simulink model "Par_model_sim_CHB7"  (R2023b)
settings: Solver=ode3  StartTime=0.0  StopTime=5  FixedStep=01e-6  RelTol=1e-3
InitFcn:
  | sysinit
values from neighbouring files (symbols this model uses):
  C = 0.0234    [sysinit.m]
  f_out = frequency_out_start : frequency_out_interval : frequency_out_end    [simout_chb_par.m]    (also in simout_chbjt_par.m = frequency_modulate_start : frequency_modulate_interval : fre)
  f_switch = 250    [sysinit.m]
  fn = 50    [sysinit.m]
  L = 0.002    [sysinit.m]
  L_1 = eps    [simout_chb_par.m]    (also in simout_chbjt_par.m; sysinit.m)
  L_ori = 0.02    [sysinit.m]
  L_sec = 0.06    [sysinit.m]
  m_par = modulate_radio_start : modulate_radio_interval : modulate_radio_end    [simout_chb_par.m]
  P0 = 8e6    (= 8000000)    [sysinit.m]
  R = 1.5    [sysinit.m]
  Source_Amp = 10000    [sysinit.m]
  st = 1e-6    (= 1e-06)    [sysinit.m]
  Td = 15e-7    (= 1.5e-06)    [sysinit.m]
  Ul_in = 1900    [sysinit.m]
libraries: spsSeriesRLCBranchLib x120, spsDiodeLib x45, spsIGBTLib x36, spsCurrentMeasurementLib x15, spsThreePhaseVIMeasurementLib x10, spsOnDelayLib x9, spsMultiWindingTransformerLib x9, spsUniversalBridgeLib x9, spsVoltageMeasurementLib x5, simulink x3, spsRMSLib x2, spsThreePhaseProgrammableVoltageSourceLib x1
(part 2 of 2)

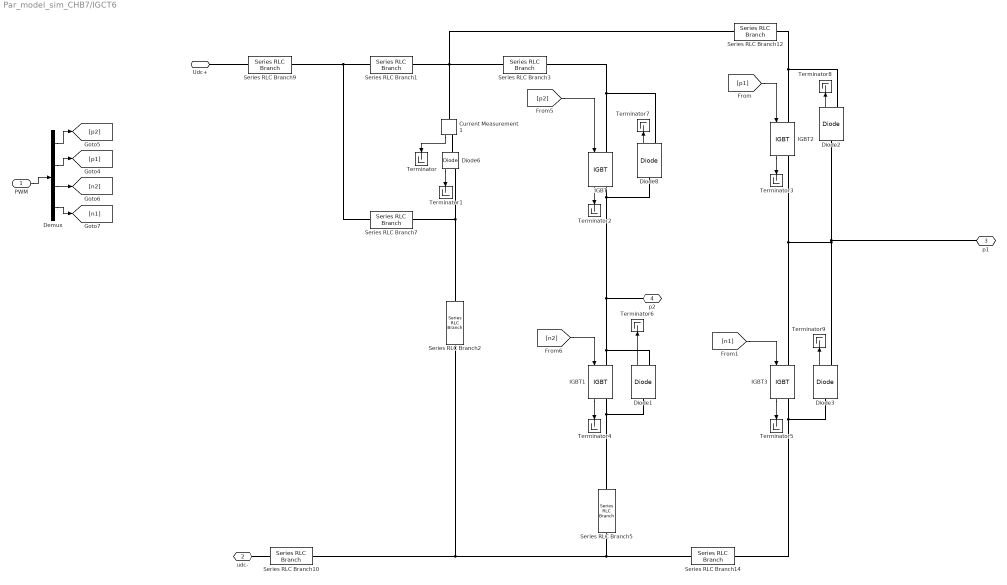
== system Par_model_sim_CHB7/IGCT6 ==
  PWM : Inport
  Current Measurement1 : spsCurrentMeasurementLib/Current Measurement  PhasorSimulation=off  OutputType=Complex  PSBequivalent=0
  Demux : Demux
  Diode{1..3,6,8} (5 alike) : spsDiodeLib/Diode  Ron=rto  Lon=0  Vf=vto  IC=0  UseSnubber=off  Rs=500  Cs=250e-9  Measurements=on
  IGBT{,1..3} (4 alike) : spsIGBTLib/IGBT  Ron=rt  Lon=0  Vf=vt  Tf=1e-6  Tt=2e-6  IC=0  Rs=1e5  Cs=inf  Measurements=on
  Series RLC Branch1 : spsSeriesRLCBranchLib/Series RLC Branch  LConnTagsString=__new0  RConnTagsString=__new0  BranchType=RL  Resistance=1e-5  Inductance=3.0E-6  SetiL0=off  InitialCurrent=0  Capacitance=1e-6  Setx0=off  InitialVoltage=0  Measurements=None
  Series RLC Branch10 : spsSeriesRLCBranchLib/Series RLC Branch  LConnTagsString=__new0  RConnTagsString=__new0  BranchType=L  Resistance=1  Inductance=0.4e-6  SetiL0=off  InitialCurrent=0  Capacitance=1e-6  Setx0=off  InitialVoltage=0  Measurements=None
  Series RLC Branch12 : spsSeriesRLCBranchLib/Series RLC Branch  LConnTagsString=__new0  RConnTagsString=__new0  BranchType=RL  Resistance=1e-5  Inductance=1E-9  SetiL0=off  InitialCurrent=0  Capacitance=1e-6  Setx0=off  InitialVoltage=0  Measurements=None
  Series RLC Branch14 : spsSeriesRLCBranchLib/Series RLC Branch  LConnTagsString=__new0  RConnTagsString=__new0  BranchType=L  Resistance=1  Inductance=1E-7  SetiL0=off  InitialCurrent=0  Capacitance=1e-6  Setx0=off  InitialVoltage=0  Measurements=None
  Series RLC Branch2 : spsSeriesRLCBranchLib/Series RLC Branch  LConnTagsString=__new0  RConnTagsString=__new0  BranchType=RC  Resistance=1e-5  Inductance=20e-6  SetiL0=off  InitialCurrent=0  Capacitance=17e-6  Setx0=off  InitialVoltage=0  Measurements=None
  Series RLC Branch3 : spsSeriesRLCBranchLib/Series RLC Branch  LConnTagsString=__new0  RConnTagsString=__new0  BranchType=RL  Resistance=1e-5  Inductance=1E-9  SetiL0=off  InitialCurrent=0  Capacitance=1e-6  Setx0=off  InitialVoltage=0  Measurements=None
  Series RLC Branch5 : spsSeriesRLCBranchLib/Series RLC Branch  LConnTagsString=__new0  RConnTagsString=__new0  BranchType=L  Resistance=1  Inductance=1E-7  SetiL0=off  InitialCurrent=0  Capacitance=1e-6  Setx0=off  InitialVoltage=0  Measurements=None
  Series RLC Branch7 : spsSeriesRLCBranchLib/Series RLC Branch  LConnTagsString=__new0  RConnTagsString=__new0  BranchType=RL  Resistance=0.6  Inductance=1e-6  SetiL0=off  InitialCurrent=0  Capacitance=1e-6  Setx0=off  InitialVoltage=0  Measurements=None
  Series RLC Branch9 : spsSeriesRLCBranchLib/Series RLC Branch  LConnTagsString=__new0  RConnTagsString=__new0  BranchType=L  Resistance=1  Inductance=0.4e-6  SetiL0=off  InitialCurrent=0  Capacitance=1e-6  Setx0=off  InitialVoltage=0  Measurements=None
  Terminator{,1..9} (10 alike) : Terminator
  Udc+ : PMIOPort  Side=Left
  udc- : PMIOPort  Port=2  Side=Left
  p1 : PMIOPort  Port=3  Side=Right
  p2 : PMIOPort  Port=4  Side=Right
  wires:
  Diode3/1 -> Terminator9/1
  IGBT3/1 -> Terminator5/1
  [n1] -> IGBT3/1
  IGBT1/1 -> Terminator4/1
  IGBT2/1 -> Terminator3/1
  IGBT/1 -> Terminator2/1
  [n2] -> IGBT1/1
  [p1] -> IGBT2/1
  Current Measurement1/1 -> Terminator/1
  Diode2/1 -> Terminator8/1
  [p2] -> IGBT/1
  Diode8/1 -> Terminator7/1
  Diode1/1 -> Terminator6/1
  Diode6/1 -> Terminator1/1
  Demux/3 -> [n2]
  PWM/1 -> Demux/1
  Demux/1 -> [p2]
  Demux/2 -> [p1]
  Demux/4 -> [n1]
  connections:
  Series RLC Branch10/LConn1 -- udc-/RConn1
  Series RLC Branch9/LConn1 -- Udc+/RConn1
  Diode6/RConn1 -- Series RLC Branch7/RConn1 -- Series RLC Branch2/LConn1
  Current Measurement1/LConn1 -- Series RLC Branch1/RConn1 -- Series RLC Branch3/LConn1 -- Series RLC Branch12/LConn1
  Diode3/LConn1 -- IGBT3/RConn1 -- Series RLC Branch14/RConn1
  Series RLC Branch3/RConn1 -- IGBT/LConn1 -- Diode8/RConn1
  Diode1/LConn1 -- Series RLC Branch5/RConn1 -- IGBT1/RConn1
  Current Measurement1/RConn1 -- Diode6/LConn1
  Diode2/RConn1 -- Series RLC Branch12/RConn1 -- IGBT2/LConn1
  p1/RConn1 -- Diode2/LConn1 -- Diode3/RConn1 -- IGBT3/LConn1 -- IGBT2/RConn1
  Series RLC Branch5/LConn1 -- Series RLC Branch14/LConn1 -- Series RLC Branch10/RConn1 -- Series RLC Branch2/RConn1
  Series RLC Branch1/LConn1 -- Series RLC Branch7/LConn1 -- Series RLC Branch9/RConn1
  p2/RConn1 -- IGBT1/LConn1 -- Diode1/RConn1 -- Diode8/LConn1 -- IGBT/RConn1

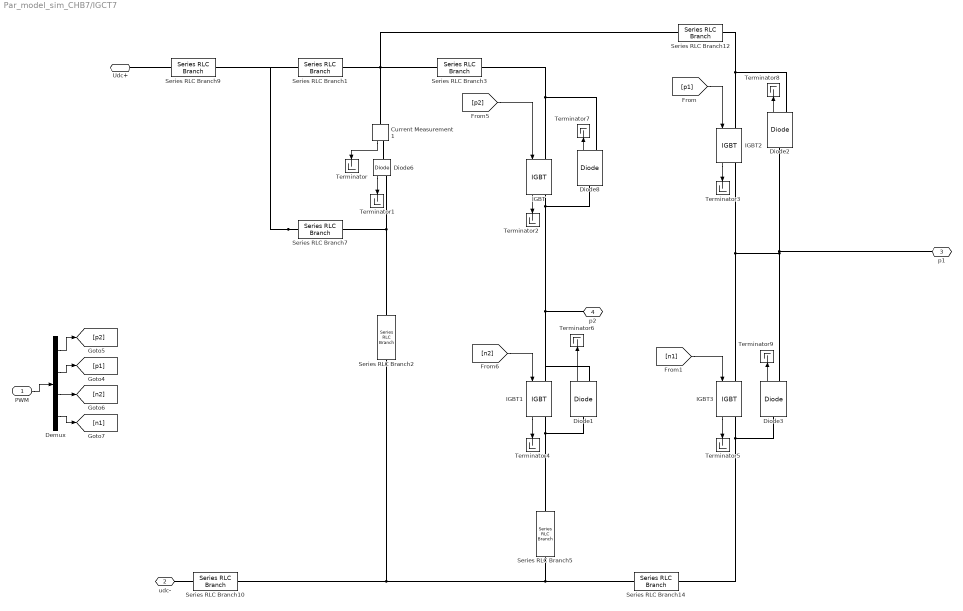
== system Par_model_sim_CHB7/IGCT7 ==
  PWM : Inport
  Current Measurement1 : spsCurrentMeasurementLib/Current Measurement  PhasorSimulation=off  OutputType=Complex  PSBequivalent=0
  Demux : Demux
  Diode{1..3,6,8} (5 alike) : spsDiodeLib/Diode  Ron=rto  Lon=0  Vf=vto  IC=0  UseSnubber=off  Rs=500  Cs=250e-9  Measurements=on
  IGBT{,1..3} (4 alike) : spsIGBTLib/IGBT  Ron=rt  Lon=0  Vf=vt  Tf=1e-6  Tt=2e-6  IC=0  Rs=1e5  Cs=inf  Measurements=on
  Series RLC Branch1 : spsSeriesRLCBranchLib/Series RLC Branch  LConnTagsString=__new0  RConnTagsString=__new0  BranchType=RL  Resistance=1e-5  Inductance=3.0E-6  SetiL0=off  InitialCurrent=0  Capacitance=1e-6  Setx0=off  InitialVoltage=0  Measurements=None
  Series RLC Branch10 : spsSeriesRLCBranchLib/Series RLC Branch  LConnTagsString=__new0  RConnTagsString=__new0  BranchType=L  Resistance=1  Inductance=0.4e-6  SetiL0=off  InitialCurrent=0  Capacitance=1e-6  Setx0=off  InitialVoltage=0  Measurements=None
  Series RLC Branch12 : spsSeriesRLCBranchLib/Series RLC Branch  LConnTagsString=__new0  RConnTagsString=__new0  BranchType=RL  Resistance=1e-5  Inductance=1E-9  SetiL0=off  InitialCurrent=0  Capacitance=1e-6  Setx0=off  InitialVoltage=0  Measurements=None
  Series RLC Branch14 : spsSeriesRLCBranchLib/Series RLC Branch  LConnTagsString=__new0  RConnTagsString=__new0  BranchType=L  Resistance=1  Inductance=1E-7  SetiL0=off  InitialCurrent=0  Capacitance=1e-6  Setx0=off  InitialVoltage=0  Measurements=None
  Series RLC Branch2 : spsSeriesRLCBranchLib/Series RLC Branch  LConnTagsString=__new0  RConnTagsString=__new0  BranchType=RC  Resistance=1e-5  Inductance=20e-6  SetiL0=off  InitialCurrent=0  Capacitance=17e-6  Setx0=off  InitialVoltage=0  Measurements=None
  Series RLC Branch3 : spsSeriesRLCBranchLib/Series RLC Branch  LConnTagsString=__new0  RConnTagsString=__new0  BranchType=RL  Resistance=1e-5  Inductance=1E-9  SetiL0=off  InitialCurrent=0  Capacitance=1e-6  Setx0=off  InitialVoltage=0  Measurements=None
  Series RLC Branch5 : spsSeriesRLCBranchLib/Series RLC Branch  LConnTagsString=__new0  RConnTagsString=__new0  BranchType=L  Resistance=1  Inductance=1E-7  SetiL0=off  InitialCurrent=0  Capacitance=1e-6  Setx0=off  InitialVoltage=0  Measurements=None
  Series RLC Branch7 : spsSeriesRLCBranchLib/Series RLC Branch  LConnTagsString=__new0  RConnTagsString=__new0  BranchType=RL  Resistance=0.6  Inductance=1e-6  SetiL0=off  InitialCurrent=0  Capacitance=1e-6  Setx0=off  InitialVoltage=0  Measurements=None
  Series RLC Branch9 : spsSeriesRLCBranchLib/Series RLC Branch  LConnTagsString=__new0  RConnTagsString=__new0  BranchType=L  Resistance=1  Inductance=0.4e-6  SetiL0=off  InitialCurrent=0  Capacitance=1e-6  Setx0=off  InitialVoltage=0  Measurements=None
  Terminator{,1..9} (10 alike) : Terminator
  Udc+ : PMIOPort  Side=Left
  udc- : PMIOPort  Port=2  Side=Left
  p1 : PMIOPort  Port=3  Side=Right
  p2 : PMIOPort  Port=4  Side=Right
  wires:
  Diode6/1 -> Terminator1/1
  Diode1/1 -> Terminator6/1
  Diode8/1 -> Terminator7/1
  PWM/1 -> Demux/1
  [p2] -> IGBT/1
  Diode2/1 -> Terminator8/1
  Current Measurement1/1 -> Terminator/1
  [p1] -> IGBT2/1
  [n2] -> IGBT1/1
  IGBT/1 -> Terminator2/1
  IGBT2/1 -> Terminator3/1
  Demux/4 -> [n1]
  Demux/3 -> [n2]
  Demux/2 -> [p1]
  IGBT1/1 -> Terminator4/1
  [n1] -> IGBT3/1
  IGBT3/1 -> Terminator5/1
  Diode3/1 -> Terminator9/1
  Demux/1 -> [p2]
  connections:
  IGBT/RConn1 -- Diode8/LConn1 -- p2/RConn1 -- Diode1/RConn1 -- IGBT1/LConn1
  Series RLC Branch7/LConn1 -- Series RLC Branch1/LConn1 -- Series RLC Branch9/RConn1
  Series RLC Branch14/LConn1 -- Series RLC Branch2/RConn1 -- Series RLC Branch10/RConn1 -- Series RLC Branch5/LConn1
  Diode2/LConn1 -- IGBT2/RConn1 -- IGBT3/LConn1 -- Diode3/RConn1 -- p1/RConn1
  Series RLC Branch12/RConn1 -- IGBT2/LConn1 -- Diode2/RConn1
  Current Measurement1/RConn1 -- Diode6/LConn1
  Series RLC Branch5/RConn1 -- Diode1/LConn1 -- IGBT1/RConn1
  IGBT/LConn1 -- Diode8/RConn1 -- Series RLC Branch3/RConn1
  IGBT3/RConn1 -- Diode3/LConn1 -- Series RLC Branch14/RConn1
  Series RLC Branch1/RConn1 -- Current Measurement1/LConn1 -- Series RLC Branch12/LConn1 -- Series RLC Branch3/LConn1
  Series RLC Branch7/RConn1 -- Diode6/RConn1 -- Series RLC Branch2/LConn1
  Series RLC Branch9/LConn1 -- Udc+/RConn1
  Series RLC Branch10/LConn1 -- udc-/RConn1

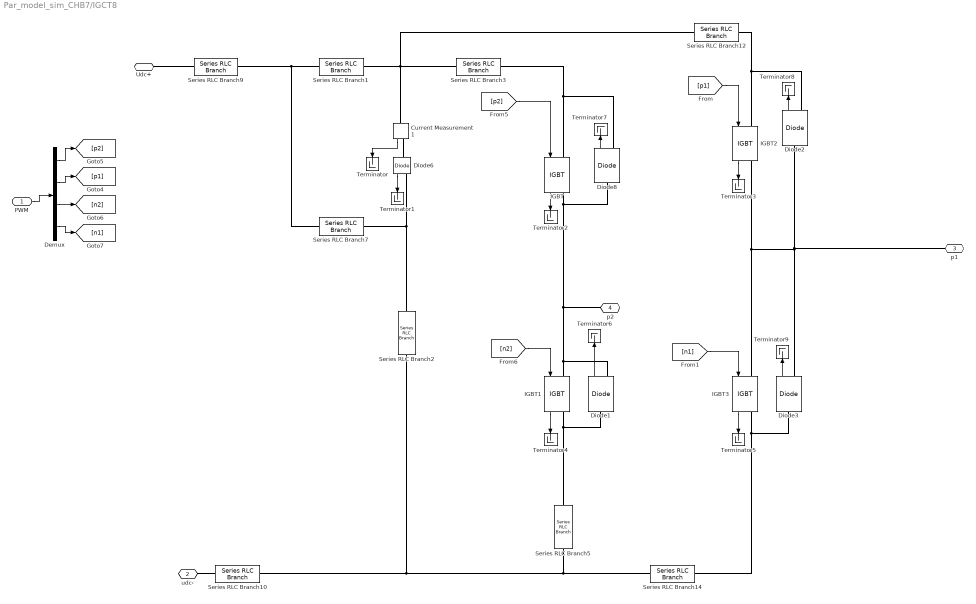
== system Par_model_sim_CHB7/IGCT8 ==
  PWM : Inport
  Current Measurement1 : spsCurrentMeasurementLib/Current Measurement  PhasorSimulation=off  OutputType=Complex  PSBequivalent=0
  Demux : Demux
  Diode{1..3,6,8} (5 alike) : spsDiodeLib/Diode  Ron=rto  Lon=0  Vf=vto  IC=0  UseSnubber=off  Rs=500  Cs=250e-9  Measurements=on
  IGBT{,1..3} (4 alike) : spsIGBTLib/IGBT  Ron=rt  Lon=0  Vf=vt  Tf=1e-6  Tt=2e-6  IC=0  Rs=1e5  Cs=inf  Measurements=on
  Series RLC Branch1 : spsSeriesRLCBranchLib/Series RLC Branch  LConnTagsString=__new0  RConnTagsString=__new0  BranchType=RL  Resistance=1e-5  Inductance=3.0E-6  SetiL0=off  InitialCurrent=0  Capacitance=1e-6  Setx0=off  InitialVoltage=0  Measurements=None
  Series RLC Branch10 : spsSeriesRLCBranchLib/Series RLC Branch  LConnTagsString=__new0  RConnTagsString=__new0  BranchType=L  Resistance=1  Inductance=0.4e-6  SetiL0=off  InitialCurrent=0  Capacitance=1e-6  Setx0=off  InitialVoltage=0  Measurements=None
  Series RLC Branch12 : spsSeriesRLCBranchLib/Series RLC Branch  LConnTagsString=__new0  RConnTagsString=__new0  BranchType=RL  Resistance=1e-5  Inductance=1E-9  SetiL0=off  InitialCurrent=0  Capacitance=1e-6  Setx0=off  InitialVoltage=0  Measurements=None
  Series RLC Branch14 : spsSeriesRLCBranchLib/Series RLC Branch  LConnTagsString=__new0  RConnTagsString=__new0  BranchType=L  Resistance=1  Inductance=1E-7  SetiL0=off  InitialCurrent=0  Capacitance=1e-6  Setx0=off  InitialVoltage=0  Measurements=None
  Series RLC Branch2 : spsSeriesRLCBranchLib/Series RLC Branch  LConnTagsString=__new0  RConnTagsString=__new0  BranchType=RC  Resistance=1e-5  Inductance=20e-6  SetiL0=off  InitialCurrent=0  Capacitance=17e-6  Setx0=off  InitialVoltage=0  Measurements=None
  Series RLC Branch3 : spsSeriesRLCBranchLib/Series RLC Branch  LConnTagsString=__new0  RConnTagsString=__new0  BranchType=RL  Resistance=1e-5  Inductance=1E-9  SetiL0=off  InitialCurrent=0  Capacitance=1e-6  Setx0=off  InitialVoltage=0  Measurements=None
  Series RLC Branch5 : spsSeriesRLCBranchLib/Series RLC Branch  LConnTagsString=__new0  RConnTagsString=__new0  BranchType=L  Resistance=1  Inductance=1E-7  SetiL0=off  InitialCurrent=0  Capacitance=1e-6  Setx0=off  InitialVoltage=0  Measurements=None
  Series RLC Branch7 : spsSeriesRLCBranchLib/Series RLC Branch  LConnTagsString=__new0  RConnTagsString=__new0  BranchType=RL  Resistance=0.6  Inductance=1e-6  SetiL0=off  InitialCurrent=0  Capacitance=1e-6  Setx0=off  InitialVoltage=0  Measurements=None
  Series RLC Branch9 : spsSeriesRLCBranchLib/Series RLC Branch  LConnTagsString=__new0  RConnTagsString=__new0  BranchType=L  Resistance=1  Inductance=0.4e-6  SetiL0=off  InitialCurrent=0  Capacitance=1e-6  Setx0=off  InitialVoltage=0  Measurements=None
  Terminator{,1..9} (10 alike) : Terminator
  Udc+ : PMIOPort  Side=Left
  udc- : PMIOPort  Port=2  Side=Left
  p1 : PMIOPort  Port=3  Side=Right
  p2 : PMIOPort  Port=4  Side=Right
  wires:
  Diode3/1 -> Terminator9/1
  IGBT3/1 -> Terminator5/1
  [n1] -> IGBT3/1
  IGBT1/1 -> Terminator4/1
  IGBT2/1 -> Terminator3/1
  IGBT/1 -> Terminator2/1
  [n2] -> IGBT1/1
  [p1] -> IGBT2/1
  Current Measurement1/1 -> Terminator/1
  Diode2/1 -> Terminator8/1
  [p2] -> IGBT/1
  Diode8/1 -> Terminator7/1
  Diode1/1 -> Terminator6/1
  Diode6/1 -> Terminator1/1
  Demux/3 -> [n2]
  PWM/1 -> Demux/1
  Demux/1 -> [p2]
  Demux/2 -> [p1]
  Demux/4 -> [n1]
  connections:
  Series RLC Branch10/LConn1 -- udc-/RConn1
  Series RLC Branch9/LConn1 -- Udc+/RConn1
  Diode6/RConn1 -- Series RLC Branch7/RConn1 -- Series RLC Branch2/LConn1
  Current Measurement1/LConn1 -- Series RLC Branch1/RConn1 -- Series RLC Branch3/LConn1 -- Series RLC Branch12/LConn1
  Diode3/LConn1 -- IGBT3/RConn1 -- Series RLC Branch14/RConn1
  Series RLC Branch3/RConn1 -- IGBT/LConn1 -- Diode8/RConn1
  Diode1/LConn1 -- Series RLC Branch5/RConn1 -- IGBT1/RConn1
  Current Measurement1/RConn1 -- Diode6/LConn1
  Diode2/RConn1 -- Series RLC Branch12/RConn1 -- IGBT2/LConn1
  p1/RConn1 -- Diode2/LConn1 -- Diode3/RConn1 -- IGBT3/LConn1 -- IGBT2/RConn1
  Series RLC Branch5/LConn1 -- Series RLC Branch14/LConn1 -- Series RLC Branch10/RConn1 -- Series RLC Branch2/RConn1
  Series RLC Branch1/LConn1 -- Series RLC Branch7/LConn1 -- Series RLC Branch9/RConn1
  p2/RConn1 -- IGBT1/LConn1 -- Diode1/RConn1 -- Diode8/LConn1 -- IGBT/RConn1

== system Par_model_sim_CHB7/IGCT9 ==
  PWM : Inport
  Current Measurement1 : spsCurrentMeasurementLib/Current Measurement  PhasorSimulation=off  OutputType=Complex  PSBequivalent=0
  Demux : Demux
  Diode{1..3,6,8} (5 alike) : spsDiodeLib/Diode  Ron=rto  Lon=0  Vf=vto  IC=0  UseSnubber=off  Rs=500  Cs=250e-9  Measurements=on
  IGBT{,1..3} (4 alike) : spsIGBTLib/IGBT  Ron=rt  Lon=0  Vf=vt  Tf=1e-6  Tt=2e-6  IC=0  Rs=1e5  Cs=inf  Measurements=on
  Series RLC Branch1 : spsSeriesRLCBranchLib/Series RLC Branch  LConnTagsString=__new0  RConnTagsString=__new0  BranchType=RL  Resistance=1e-5  Inductance=3.0E-6  SetiL0=off  InitialCurrent=0  Capacitance=1e-6  Setx0=off  InitialVoltage=0  Measurements=None
  Series RLC Branch10 : spsSeriesRLCBranchLib/Series RLC Branch  LConnTagsString=__new0  RConnTagsString=__new0  BranchType=L  Resistance=1  Inductance=0.4e-6  SetiL0=off  InitialCurrent=0  Capacitance=1e-6  Setx0=off  InitialVoltage=0  Measurements=None
  Series RLC Branch12 : spsSeriesRLCBranchLib/Series RLC Branch  LConnTagsString=__new0  RConnTagsString=__new0  BranchType=RL  Resistance=1e-5  Inductance=1E-9  SetiL0=off  InitialCurrent=0  Capacitance=1e-6  Setx0=off  InitialVoltage=0  Measurements=None
  Series RLC Branch14 : spsSeriesRLCBranchLib/Series RLC Branch  LConnTagsString=__new0  RConnTagsString=__new0  BranchType=L  Resistance=1  Inductance=1E-7  SetiL0=off  InitialCurrent=0  Capacitance=1e-6  Setx0=off  InitialVoltage=0  Measurements=None
  Series RLC Branch2 : spsSeriesRLCBranchLib/Series RLC Branch  LConnTagsString=__new0  RConnTagsString=__new0  BranchType=RC  Resistance=1e-5  Inductance=20e-6  SetiL0=off  InitialCurrent=0  Capacitance=17e-6  Setx0=off  InitialVoltage=0  Measurements=None
  Series RLC Branch3 : spsSeriesRLCBranchLib/Series RLC Branch  LConnTagsString=__new0  RConnTagsString=__new0  BranchType=RL  Resistance=1e-5  Inductance=1E-9  SetiL0=off  InitialCurrent=0  Capacitance=1e-6  Setx0=off  InitialVoltage=0  Measurements=None
  Series RLC Branch5 : spsSeriesRLCBranchLib/Series RLC Branch  LConnTagsString=__new0  RConnTagsString=__new0  BranchType=L  Resistance=1  Inductance=1E-7  SetiL0=off  InitialCurrent=0  Capacitance=1e-6  Setx0=off  InitialVoltage=0  Measurements=None
  Series RLC Branch7 : spsSeriesRLCBranchLib/Series RLC Branch  LConnTagsString=__new0  RConnTagsString=__new0  BranchType=RL  Resistance=0.6  Inductance=1e-6  SetiL0=off  InitialCurrent=0  Capacitance=1e-6  Setx0=off  InitialVoltage=0  Measurements=None
  Series RLC Branch9 : spsSeriesRLCBranchLib/Series RLC Branch  LConnTagsString=__new0  RConnTagsString=__new0  BranchType=L  Resistance=1  Inductance=0.4e-6  SetiL0=off  InitialCurrent=0  Capacitance=1e-6  Setx0=off  InitialVoltage=0  Measurements=None
  Terminator{,1..9} (10 alike) : Terminator
  Udc+ : PMIOPort  Side=Left
  udc- : PMIOPort  Port=2  Side=Left
  p1 : PMIOPort  Port=3  Side=Right
  p2 : PMIOPort  Port=4  Side=Right
  wires:
  Diode3/1 -> Terminator9/1
  IGBT3/1 -> Terminator5/1
  [n1] -> IGBT3/1
  IGBT1/1 -> Terminator4/1
  IGBT2/1 -> Terminator3/1
  IGBT/1 -> Terminator2/1
  [n2] -> IGBT1/1
  [p1] -> IGBT2/1
  Current Measurement1/1 -> Terminator/1
  Diode2/1 -> Terminator8/1
  [p2] -> IGBT/1
  Diode8/1 -> Terminator7/1
  Diode1/1 -> Terminator6/1
  Diode6/1 -> Terminator1/1
  Demux/3 -> [n2]
  PWM/1 -> Demux/1
  Demux/1 -> [p2]
  Demux/2 -> [p1]
  Demux/4 -> [n1]
  connections:
  Series RLC Branch10/LConn1 -- udc-/RConn1
  Series RLC Branch9/LConn1 -- Udc+/RConn1
  Diode6/RConn1 -- Series RLC Branch7/RConn1 -- Series RLC Branch2/LConn1
  Current Measurement1/LConn1 -- Series RLC Branch1/RConn1 -- Series RLC Branch3/LConn1 -- Series RLC Branch12/LConn1
  Diode3/LConn1 -- IGBT3/RConn1 -- Series RLC Branch14/RConn1
  Series RLC Branch3/RConn1 -- IGBT/LConn1 -- Diode8/RConn1
  Diode1/LConn1 -- Series RLC Branch5/RConn1 -- IGBT1/RConn1
  Current Measurement1/RConn1 -- Diode6/LConn1
  Diode2/RConn1 -- Series RLC Branch12/RConn1 -- IGBT2/LConn1
  p1/RConn1 -- Diode2/LConn1 -- Diode3/RConn1 -- IGBT3/LConn1 -- IGBT2/RConn1
  Series RLC Branch5/LConn1 -- Series RLC Branch14/LConn1 -- Series RLC Branch10/RConn1 -- Series RLC Branch2/RConn1
  Series RLC Branch1/LConn1 -- Series RLC Branch7/LConn1 -- Series RLC Branch9/RConn1
  p2/RConn1 -- IGBT1/LConn1 -- Diode1/RConn1 -- Diode8/LConn1 -- IGBT/RConn1

== system Par_model_sim_CHB7/LOAD ==
  Series RLC Branch1 : spsSeriesRLCBranchLib/Series RLC Branch  LConnTagsString=__new0  RConnTagsString=__new0  BranchType=RL  Resistance=R*1.5  Inductance=L*1.5  SetiL0=off  InitialCurrent=0  Capacitance=1e-6  Setx0=off  InitialVoltage=0  Measurements=None
  Series RLC Branch2 : spsSeriesRLCBranchLib/Series RLC Branch  LConnTagsString=__new0  RConnTagsString=__new0  BranchType=RL  Resistance=R*1.5  Inductance=L*1.5  SetiL0=off  InitialCurrent=0  Capacitance=1e-6  Setx0=off  InitialVoltage=0  Measurements=None
  Series RLC Branch7 : spsSeriesRLCBranchLib/Series RLC Branch  LConnTagsString=__new0  RConnTagsString=__new0  BranchType=RL  Resistance=R*1.5  Inductance=L*1.5  SetiL0=off  InitialCurrent=0  Capacitance=1e-6  Setx0=off  InitialVoltage=0  Measurements=None
  A : PMIOPort  Side=Left
  B : PMIOPort  Port=2  Side=Left
  C : PMIOPort  Port=3  Side=Left
  connections:
  Series RLC Branch7/RConn1 -- Series RLC Branch2/RConn1 -- Series RLC Branch1/RConn1
  Series RLC Branch2/LConn1 -- C/RConn1
  Series RLC Branch7/LConn1 -- A/RConn1
  Series RLC Branch1/LConn1 -- B/RConn1

== system Par_model_sim_CHB7/Subsystem ==
  Current Measurement : spsCurrentMeasurementLib/Current Measurement  PhasorSimulation=off  OutputType=Complex  PSBequivalent=0
  Voltage Measurement : spsVoltageMeasurementLib/Voltage Measurement  PhasorSimulation=off  OutputType=Complex  PSBequivalent=0
  + : PMIOPort  Side=Left
  - : PMIOPort  Port=2  Side=Left
  +OUT : PMIOPort  Port=3  Side=Right
  -OUT : PMIOPort  Port=4  Side=Right
  tag scope: Idc1=global, Udc=global
  wires:
  Voltage Measurement/1 -> [Udc]
  Current Measurement/1 -> [Idc1]
  connections:
  Voltage Measurement/LConn1 -- Current Measurement/LConn1 -- +/RConn1
  Voltage Measurement/LConn2 -- -OUT/RConn1 -- -/RConn1
  Current Measurement/RConn1 -- +OUT/RConn1

== system Par_model_sim_CHB7/Subsystem1 ==
  Current Measurement : spsCurrentMeasurementLib/Current Measurement  PhasorSimulation=off  OutputType=Complex  PSBequivalent=0
  Voltage Measurement : spsVoltageMeasurementLib/Voltage Measurement  PhasorSimulation=off  OutputType=Complex  PSBequivalent=0
  + : PMIOPort  Side=Left
  - : PMIOPort  Port=2  Side=Left
  +OUT : PMIOPort  Port=3  Side=Right
  -OUT : PMIOPort  Port=4  Side=Right
  tag scope: Idc2=global
  wires:
  Current Measurement/1 -> [Idc2]
  connections:
  Voltage Measurement/LConn1 -- +/RConn1 -- Current Measurement/LConn1
  Voltage Measurement/LConn2 -- -OUT/RConn1 -- -/RConn1
  Current Measurement/RConn1 -- +OUT/RConn1

== system Par_model_sim_CHB7/Subsystem2 ==
  Current Measurement : spsCurrentMeasurementLib/Current Measurement  PhasorSimulation=off  OutputType=Complex  PSBequivalent=0
  Voltage Measurement : spsVoltageMeasurementLib/Voltage Measurement  PhasorSimulation=off  OutputType=Complex  PSBequivalent=0
  + : PMIOPort  Side=Left
  - : PMIOPort  Port=2  Side=Left
  +OUT : PMIOPort  Port=3  Side=Right
  -OUT : PMIOPort  Port=4  Side=Right
  tag scope: Idc3=global
  wires:
  Current Measurement/1 -> [Idc3]
  connections:
  Voltage Measurement/LConn1 -- +/RConn1 -- Current Measurement/LConn1
  Voltage Measurement/LConn2 -- -OUT/RConn1 -- -/RConn1
  Current Measurement/RConn1 -- +OUT/RConn1

== system Par_model_sim_CHB7/Subsystem3 ==
  Series RLC Branch{1..9} (9 alike) : spsSeriesRLCBranchLib/Series RLC Branch  LConnTagsString=__new0  RConnTagsString=__new0  BranchType=L  Resistance=R*1.5  Inductance=L_in  SetiL0=off  InitialCurrent=0  Capacitance=1e-6  Setx0=off  InitialVoltage=0  Measurements=None
  Conn1 : PMIOPort  Side=Left
  Conn2 : PMIOPort  Port=2  Side=Right
  Conn3 : PMIOPort  Port=3  Side=Left
  Conn4 : PMIOPort  Port=4  Side=Right
  Conn5 : PMIOPort  Port=5  Side=Left
  Conn6 : PMIOPort  Port=6  Side=Right
  Conn7 : PMIOPort  Port=7  Side=Left
  Conn8 : PMIOPort  Port=8  Side=Right
  Conn9 : PMIOPort  Port=9  Side=Left
  Conn10 : PMIOPort  Port=10  Side=Right
  Conn11 : PMIOPort  Port=11  Side=Left
  Conn12 : PMIOPort  Port=12  Side=Right
  Conn13 : PMIOPort  Port=13  Side=Left
  Conn14 : PMIOPort  Port=14  Side=Right
  Conn15 : PMIOPort  Port=15  Side=Left
  Conn16 : PMIOPort  Port=16  Side=Right
  Conn17 : PMIOPort  Port=17  Side=Left
  Conn18 : PMIOPort  Port=18  Side=Right
  connections:
  Series RLC Branch3/RConn1 -- Conn8/RConn1
  Series RLC Branch3/LConn1 -- Conn7/RConn1
  Series RLC Branch7/LConn1 -- Conn1/RConn1
  Series RLC Branch7/RConn1 -- Conn2/RConn1
  Series RLC Branch1/LConn1 -- Conn3/RConn1
  Series RLC Branch2/LConn1 -- Conn5/RConn1
  Series RLC Branch4/LConn1 -- Conn9/RConn1
  Series RLC Branch5/LConn1 -- Conn11/RConn1
  Series RLC Branch4/RConn1 -- Conn10/RConn1
  Series RLC Branch1/RConn1 -- Conn4/RConn1
  Series RLC Branch5/RConn1 -- Conn12/RConn1
  Series RLC Branch9/LConn1 -- Conn17/RConn1
  Series RLC Branch8/LConn1 -- Conn15/RConn1
  Series RLC Branch6/RConn1 -- Conn14/RConn1
  Series RLC Branch9/RConn1 -- Conn18/RConn1
  Series RLC Branch8/RConn1 -- Conn16/RConn1
  Series RLC Branch6/LConn1 -- Conn13/RConn1
  Series RLC Branch2/RConn1 -- Conn6/RConn1

== system Par_model_sim_CHB7/Subsystem4 ==
  Series RLC Branch{1..9} (9 alike) : spsSeriesRLCBranchLib/Series RLC Branch  LConnTagsString=__new0  RConnTagsString=__new0  BranchType=L  Resistance=R*1.5  Inductance=L_in  SetiL0=off  InitialCurrent=0  Capacitance=1e-6  Setx0=off  InitialVoltage=0  Measurements=None
  Conn1 : PMIOPort  Side=Left
  Conn2 : PMIOPort  Port=2  Side=Right
  Conn3 : PMIOPort  Port=3  Side=Left
  Conn4 : PMIOPort  Port=4  Side=Right
  Conn5 : PMIOPort  Port=5  Side=Left
  Conn6 : PMIOPort  Port=6  Side=Right
  Conn7 : PMIOPort  Port=7  Side=Left
  Conn8 : PMIOPort  Port=8  Side=Right
  Conn9 : PMIOPort  Port=9  Side=Left
  Conn10 : PMIOPort  Port=10  Side=Right
  Conn11 : PMIOPort  Port=11  Side=Left
  Conn12 : PMIOPort  Port=12  Side=Right
  Conn13 : PMIOPort  Port=13  Side=Left
  Conn14 : PMIOPort  Port=14  Side=Right
  Conn15 : PMIOPort  Port=15  Side=Left
  Conn16 : PMIOPort  Port=16  Side=Right
  Conn17 : PMIOPort  Port=17  Side=Left
  Conn18 : PMIOPort  Port=18  Side=Right
  connections:
  Series RLC Branch2/RConn1 -- Conn6/RConn1
  Series RLC Branch6/LConn1 -- Conn13/RConn1
  Series RLC Branch8/RConn1 -- Conn16/RConn1
  Series RLC Branch9/RConn1 -- Conn18/RConn1
  Series RLC Branch6/RConn1 -- Conn14/RConn1
  Series RLC Branch8/LConn1 -- Conn15/RConn1
  Series RLC Branch9/LConn1 -- Conn17/RConn1
  Series RLC Branch5/RConn1 -- Conn12/RConn1
  Series RLC Branch1/RConn1 -- Conn4/RConn1
  Series RLC Branch4/RConn1 -- Conn10/RConn1
  Series RLC Branch5/LConn1 -- Conn11/RConn1
  Series RLC Branch4/LConn1 -- Conn9/RConn1
  Series RLC Branch2/LConn1 -- Conn5/RConn1
  Series RLC Branch1/LConn1 -- Conn3/RConn1
  Series RLC Branch7/RConn1 -- Conn2/RConn1
  Series RLC Branch7/LConn1 -- Conn1/RConn1
  Series RLC Branch3/LConn1 -- Conn7/RConn1
  Series RLC Branch3/RConn1 -- Conn8/RConn1

== system Par_model_sim_CHB7/Subsystem5 ==
  Series RLC Branch{1..9} (9 alike) : spsSeriesRLCBranchLib/Series RLC Branch  LConnTagsString=__new0  RConnTagsString=__new0  BranchType=L  Resistance=R*1.5  Inductance=L_in  SetiL0=off  InitialCurrent=0  Capacitance=1e-6  Setx0=off  InitialVoltage=0  Measurements=None
  Conn1 : PMIOPort  Side=Left
  Conn2 : PMIOPort  Port=2  Side=Right
  Conn3 : PMIOPort  Port=3  Side=Left
  Conn4 : PMIOPort  Port=4  Side=Right
  Conn5 : PMIOPort  Port=5  Side=Left
  Conn6 : PMIOPort  Port=6  Side=Right
  Conn7 : PMIOPort  Port=7  Side=Left
  Conn8 : PMIOPort  Port=8  Side=Right
  Conn9 : PMIOPort  Port=9  Side=Left
  Conn10 : PMIOPort  Port=10  Side=Right
  Conn11 : PMIOPort  Port=11  Side=Left
  Conn12 : PMIOPort  Port=12  Side=Right
  Conn13 : PMIOPort  Port=13  Side=Left
  Conn14 : PMIOPort  Port=14  Side=Right
  Conn15 : PMIOPort  Port=15  Side=Left
  Conn16 : PMIOPort  Port=16  Side=Right
  Conn17 : PMIOPort  Port=17  Side=Left
  Conn18 : PMIOPort  Port=18  Side=Right
  connections:
  Series RLC Branch3/RConn1 -- Conn8/RConn1
  Series RLC Branch3/LConn1 -- Conn7/RConn1
  Series RLC Branch7/LConn1 -- Conn1/RConn1
  Series RLC Branch7/RConn1 -- Conn2/RConn1
  Series RLC Branch1/LConn1 -- Conn3/RConn1
  Series RLC Branch2/LConn1 -- Conn5/RConn1
  Series RLC Branch4/LConn1 -- Conn9/RConn1
  Series RLC Branch5/LConn1 -- Conn11/RConn1
  Series RLC Branch4/RConn1 -- Conn10/RConn1
  Series RLC Branch1/RConn1 -- Conn4/RConn1
  Series RLC Branch5/RConn1 -- Conn12/RConn1
  Series RLC Branch9/LConn1 -- Conn17/RConn1
  Series RLC Branch8/LConn1 -- Conn15/RConn1
  Series RLC Branch6/RConn1 -- Conn14/RConn1
  Series RLC Branch9/RConn1 -- Conn18/RConn1
  Series RLC Branch8/RConn1 -- Conn16/RConn1
  Series RLC Branch6/LConn1 -- Conn13/RConn1
  Series RLC Branch2/RConn1 -- Conn6/RConn1

== system Par_model_sim_CHB7/Subsystem6 ==
  Multi-Winding Transformer10 : spsMultiWindingTransformerLib/Multi-Winding Transformer  LeftWindings=1  RightWindings=5  TappedWindings=no taps  NumberOfTaps=2  SetSaturation=off  Hysteresis=off  DataFile='hysteresis.mat'  Measurements=None  UNITS=pu  NominalPower=[P0 fn]  NominalVoltages="[ Source_Amp   (1-sin(10/180*pi)/sin(50/180*pi))*2*sin(50/180*pi)*Ul_in sin(10/180*pi)/sin(50/180*pi)*2*sin(50/180*pi)*Ul_in  Ul_in (1-sin(10/180*pi)/sin(50/180*pi))*2*sin(50/180*pi)*Ul_in sin(10/180*pi)/sin(50/180*pi)*2*sin(50/180*pi)*Ul_in]"  WindingResistances="[ 0.005   0.005 0.005 0.005  0.005  0.005]"  WindingInductances="[ L_ori*5  L_sec L_sec L_sec L_sec L_sec]/5"  Rm=50  Lm=50  Saturation=[ 0,0 ; 0.0024,1.2 ; 1.0,1.52 ]  SpecifyInitialFlux=off  InitialFlux=0  BreakLoop=off  DiscreteSolver=Trapezoidal iterative  DataType=off  TransfoNumber=1
      settings: LibrarySourceBlock=|
      | sps_lib/Power Grid Elements/Multi-Winding
      | Transformer
  Multi-Winding Transformer11 : spsMultiWindingTransformerLib/Multi-Winding Transformer  LeftWindings=1  RightWindings=5  TappedWindings=no taps  NumberOfTaps=2  SetSaturation=off  Hysteresis=off  DataFile='hysteresis.mat'  Measurements=None  UNITS=pu  NominalPower=[P0 fn]  NominalVoltages="[ Source_Amp   (1-sin(10/180*pi)/sin(50/180*pi))*2*sin(50/180*pi)*Ul_in sin(10/180*pi)/sin(50/180*pi)*2*sin(50/180*pi)*Ul_in  Ul_in (1-sin(10/180*pi)/sin(50/180*pi))*2*sin(50/180*pi)*Ul_in sin(10/180*pi)/sin(50/180*pi)*2*sin(50/180*pi)*Ul_in]"  WindingResistances="[ 0.005   0.005 0.005 0.005  0.005  0.005]"  WindingInductances="[ L_ori*5  L_sec L_sec L_sec L_sec L_sec]/5"  Rm=50  Lm=50  Saturation=[ 0,0 ; 0.0024,1.2 ; 1.0,1.52 ]  SpecifyInitialFlux=off  InitialFlux=0  BreakLoop=off  DiscreteSolver=Trapezoidal iterative  DataType=off  TransfoNumber=1
      settings: LibrarySourceBlock=|
      | sps_lib/Power Grid Elements/Multi-Winding
      | Transformer
  Multi-Winding Transformer9 : spsMultiWindingTransformerLib/Multi-Winding Transformer  LeftWindings=1  RightWindings=5  TappedWindings=no taps  NumberOfTaps=2  SetSaturation=off  Hysteresis=off  DataFile='hysteresis.mat'  Measurements=None  UNITS=pu  NominalPower=[P0 fn]  NominalVoltages="[ Source_Amp (1-sin(10/180*pi)/sin(50/180*pi))*2*sin(50/180*pi)*Ul_in sin(10/180*pi)/sin(50/180*pi)*2*sin(50/180*pi)*Ul_in  Ul_in (1-sin(10/180*pi)/sin(50/180*pi))*2*sin(50/180*pi)*Ul_in sin(10/180*pi)/sin(50/180*pi)*2*sin(50/180*pi)*Ul_in]"  WindingResistances="[ 0.005   0.005 0.005 0.005  0.005  0.005]"  WindingInductances="[ L_ori*5  L_sec L_sec L_sec L_sec L_sec]/5"  Rm=50  Lm=50  Saturation=[ 0,0 ; 0.0024,1.2 ; 1.0,1.52 ]  SpecifyInitialFlux=off  InitialFlux=0  BreakLoop=off  DiscreteSolver=Trapezoidal iterative  DataType=off  TransfoNumber=1
      settings: LibrarySourceBlock=|
      | sps_lib/Power Grid Elements/Multi-Winding
      | Transformer
  1+ : PMIOPort  Side=Left
  1+1 : PMIOPort  Port=2  Side=Left
  1+2 : PMIOPort  Port=3  Side=Left
  -20a : PMIOPort  Port=4  Side=Right
  -20b : PMIOPort  Port=5  Side=Right
  -20c : PMIOPort  Port=6  Side=Right
  0a : PMIOPort  Port=7  Side=Right
  0b : PMIOPort  Port=8  Side=Right
  0c : PMIOPort  Port=9  Side=Right
  +20a : PMIOPort  Port=10  Side=Right
  +20b : PMIOPort  Port=11  Side=Right
  +20c : PMIOPort  Port=12  Side=Right
  connections:
  Multi-Winding Transformer10/RConn9 -- +20b/RConn1
  Multi-Winding Transformer10/RConn5 -- 0b/RConn1
  Multi-Winding Transformer9/LConn1 -- 1+/RConn1
  Multi-Winding Transformer11/RConn9 -- +20c/RConn1
  +20a/RConn1 -- Multi-Winding Transformer9/RConn9
  Multi-Winding Transformer10/LConn1 -- 1+1/RConn1
  Multi-Winding Transformer9/RConn5 -- 0a/RConn1
  -20a/RConn1 -- Multi-Winding Transformer9/RConn3
  Multi-Winding Transformer11/RConn5 -- 0c/RConn1
  Multi-Winding Transformer11/LConn1 -- 1+2/RConn1
  Multi-Winding Transformer11/RConn3 -- -20c/RConn1
  Multi-Winding Transformer11/RConn2 -- Multi-Winding Transformer10/RConn4 -- Multi-Winding Transformer10/RConn1
  Multi-Winding Transformer10/RConn3 -- -20b/RConn1
  Multi-Winding Transformer11/RConn8 -- Multi-Winding Transformer9/RConn7 -- Multi-Winding Transformer9/RConn10
  Multi-Winding Transformer11/RConn4 -- Multi-Winding Transformer9/RConn2 -- Multi-Winding Transformer11/RConn1
  Multi-Winding Transformer10/RConn10 -- Multi-Winding Transformer9/RConn8 -- Multi-Winding Transformer10/RConn7
  Multi-Winding Transformer11/RConn6 -- Multi-Winding Transformer9/RConn6 -- Multi-Winding Transformer10/RConn6
  Multi-Winding Transformer10/RConn2 -- Multi-Winding Transformer9/RConn4 -- Multi-Winding Transformer9/RConn1
  Multi-Winding Transformer11/RConn10 -- Multi-Winding Transformer10/RConn8 -- Multi-Winding Transformer11/RConn7
  Multi-Winding Transformer11/LConn2 -- Multi-Winding Transformer9/LConn2 -- Multi-Winding Transformer10/LConn2

== system Par_model_sim_CHB7/Subsystem7 ==
  Multi-Winding Transformer10 : spsMultiWindingTransformerLib/Multi-Winding Transformer  LeftWindings=1  RightWindings=5  TappedWindings=no taps  NumberOfTaps=2  SetSaturation=off  Hysteresis=off  DataFile='hysteresis.mat'  Measurements=None  UNITS=pu  NominalPower=[P0 fn]  NominalVoltages="[ Source_Amp   (1-sin(10/180*pi)/sin(50/180*pi))*2*sin(50/180*pi)*Ul_in sin(10/180*pi)/sin(50/180*pi)*2*sin(50/180*pi)*Ul_in  Ul_in (1-sin(10/180*pi)/sin(50/180*pi))*2*sin(50/180*pi)*Ul_in sin(10/180*pi)/sin(50/180*pi)*2*sin(50/180*pi)*Ul_in]"  WindingResistances="[ 0.005   0.005 0.005 0.005  0.005  0.005]"  WindingInductances="[ L_ori*5  L_sec L_sec L_sec L_sec L_sec]/5"  Rm=50  Lm=50  Saturation=[ 0,0 ; 0.0024,1.2 ; 1.0,1.52 ]  SpecifyInitialFlux=off  InitialFlux=0  BreakLoop=off  DiscreteSolver=Trapezoidal iterative  DataType=off  TransfoNumber=1
      settings: LibrarySourceBlock=|
      | sps_lib/Power Grid Elements/Multi-Winding
      | Transformer
  Multi-Winding Transformer11 : spsMultiWindingTransformerLib/Multi-Winding Transformer  LeftWindings=1  RightWindings=5  TappedWindings=no taps  NumberOfTaps=2  SetSaturation=off  Hysteresis=off  DataFile='hysteresis.mat'  Measurements=None  UNITS=pu  NominalPower=[P0 fn]  NominalVoltages="[ Source_Amp   (1-sin(10/180*pi)/sin(50/180*pi))*2*sin(50/180*pi)*Ul_in sin(10/180*pi)/sin(50/180*pi)*2*sin(50/180*pi)*Ul_in  Ul_in (1-sin(10/180*pi)/sin(50/180*pi))*2*sin(50/180*pi)*Ul_in sin(10/180*pi)/sin(50/180*pi)*2*sin(50/180*pi)*Ul_in]"  WindingResistances="[ 0.005   0.005 0.005 0.005  0.005  0.005]"  WindingInductances="[ L_ori*5  L_sec L_sec L_sec L_sec L_sec]/5"  Rm=50  Lm=50  Saturation=[ 0,0 ; 0.0024,1.2 ; 1.0,1.52 ]  SpecifyInitialFlux=off  InitialFlux=0  BreakLoop=off  DiscreteSolver=Trapezoidal iterative  DataType=off  TransfoNumber=1
      settings: LibrarySourceBlock=|
      | sps_lib/Power Grid Elements/Multi-Winding
      | Transformer
  Multi-Winding Transformer9 : spsMultiWindingTransformerLib/Multi-Winding Transformer  LeftWindings=1  RightWindings=5  TappedWindings=no taps  NumberOfTaps=2  SetSaturation=off  Hysteresis=off  DataFile='hysteresis.mat'  Measurements=None  UNITS=pu  NominalPower=[P0 fn]  NominalVoltages="[ Source_Amp (1-sin(10/180*pi)/sin(50/180*pi))*2*sin(50/180*pi)*Ul_in sin(10/180*pi)/sin(50/180*pi)*2*sin(50/180*pi)*Ul_in  Ul_in (1-sin(10/180*pi)/sin(50/180*pi))*2*sin(50/180*pi)*Ul_in sin(10/180*pi)/sin(50/180*pi)*2*sin(50/180*pi)*Ul_in]"  WindingResistances="[ 0.005   0.005 0.005 0.005  0.005  0.005]"  WindingInductances="[ L_ori*5  L_sec L_sec L_sec L_sec L_sec]/5"  Rm=50  Lm=50  Saturation=[ 0,0 ; 0.0024,1.2 ; 1.0,1.52 ]  SpecifyInitialFlux=off  InitialFlux=0  BreakLoop=off  DiscreteSolver=Trapezoidal iterative  DataType=off  TransfoNumber=1
      settings: LibrarySourceBlock=|
      | sps_lib/Power Grid Elements/Multi-Winding
      | Transformer
  1+ : PMIOPort  Side=Left
  1+1 : PMIOPort  Port=2  Side=Left
  1+2 : PMIOPort  Port=3  Side=Left
  -20a : PMIOPort  Port=4  Side=Right
  -20b : PMIOPort  Port=5  Side=Right
  -20c : PMIOPort  Port=6  Side=Right
  0a : PMIOPort  Port=7  Side=Right
  0b : PMIOPort  Port=8  Side=Right
  0c : PMIOPort  Port=9  Side=Right
  +20a : PMIOPort  Port=10  Side=Right
  +20b : PMIOPort  Port=11  Side=Right
  +20c : PMIOPort  Port=12  Side=Right
  connections:
  Multi-Winding Transformer10/LConn2 -- Multi-Winding Transformer9/LConn2 -- Multi-Winding Transformer11/LConn2
  Multi-Winding Transformer11/RConn7 -- Multi-Winding Transformer10/RConn8 -- Multi-Winding Transformer11/RConn10
  Multi-Winding Transformer9/RConn1 -- Multi-Winding Transformer9/RConn4 -- Multi-Winding Transformer10/RConn2
  Multi-Winding Transformer10/RConn6 -- Multi-Winding Transformer9/RConn6 -- Multi-Winding Transformer11/RConn6
  Multi-Winding Transformer10/RConn7 -- Multi-Winding Transformer9/RConn8 -- Multi-Winding Transformer10/RConn10
  Multi-Winding Transformer11/RConn1 -- Multi-Winding Transformer9/RConn2 -- Multi-Winding Transformer11/RConn4
  Multi-Winding Transformer9/RConn10 -- Multi-Winding Transformer9/RConn7 -- Multi-Winding Transformer11/RConn8
  Multi-Winding Transformer10/RConn3 -- -20b/RConn1
  Multi-Winding Transformer10/RConn1 -- Multi-Winding Transformer10/RConn4 -- Multi-Winding Transformer11/RConn2
  Multi-Winding Transformer11/RConn3 -- -20c/RConn1
  Multi-Winding Transformer11/LConn1 -- 1+2/RConn1
  Multi-Winding Transformer11/RConn5 -- 0c/RConn1
  -20a/RConn1 -- Multi-Winding Transformer9/RConn3
  Multi-Winding Transformer9/RConn5 -- 0a/RConn1
  Multi-Winding Transformer10/LConn1 -- 1+1/RConn1
  +20a/RConn1 -- Multi-Winding Transformer9/RConn9
  Multi-Winding Transformer11/RConn9 -- +20c/RConn1
  Multi-Winding Transformer9/LConn1 -- 1+/RConn1
  Multi-Winding Transformer10/RConn5 -- 0b/RConn1
  Multi-Winding Transformer10/RConn9 -- +20b/RConn1

== system Par_model_sim_CHB7/Subsystem8 ==
  Multi-Winding Transformer10 : spsMultiWindingTransformerLib/Multi-Winding Transformer  LeftWindings=1  RightWindings=5  TappedWindings=no taps  NumberOfTaps=2  SetSaturation=off  Hysteresis=off  DataFile='hysteresis.mat'  Measurements=None  UNITS=pu  NominalPower=[P0 fn]  NominalVoltages="[ Source_Amp   (1-sin(10/180*pi)/sin(50/180*pi))*2*sin(50/180*pi)*Ul_in sin(10/180*pi)/sin(50/180*pi)*2*sin(50/180*pi)*Ul_in  Ul_in (1-sin(10/180*pi)/sin(50/180*pi))*2*sin(50/180*pi)*Ul_in sin(10/180*pi)/sin(50/180*pi)*2*sin(50/180*pi)*Ul_in]"  WindingResistances="[ 0.005   0.005 0.005 0.005  0.005  0.005]"  WindingInductances="[ L_ori*5  L_sec L_sec L_sec L_sec L_sec]/5"  Rm=50  Lm=50  Saturation=[ 0,0 ; 0.0024,1.2 ; 1.0,1.52 ]  SpecifyInitialFlux=off  InitialFlux=0  BreakLoop=off  DiscreteSolver=Trapezoidal iterative  DataType=off  TransfoNumber=1
      settings: LibrarySourceBlock=|
      | sps_lib/Power Grid Elements/Multi-Winding
      | Transformer
  Multi-Winding Transformer11 : spsMultiWindingTransformerLib/Multi-Winding Transformer  LeftWindings=1  RightWindings=5  TappedWindings=no taps  NumberOfTaps=2  SetSaturation=off  Hysteresis=off  DataFile='hysteresis.mat'  Measurements=None  UNITS=pu  NominalPower=[P0 fn]  NominalVoltages="[ Source_Amp   (1-sin(10/180*pi)/sin(50/180*pi))*2*sin(50/180*pi)*Ul_in sin(10/180*pi)/sin(50/180*pi)*2*sin(50/180*pi)*Ul_in  Ul_in (1-sin(10/180*pi)/sin(50/180*pi))*2*sin(50/180*pi)*Ul_in sin(10/180*pi)/sin(50/180*pi)*2*sin(50/180*pi)*Ul_in]"  WindingResistances="[ 0.005   0.005 0.005 0.005  0.005  0.005]"  WindingInductances="[ L_ori*5  L_sec L_sec L_sec L_sec L_sec]/5"  Rm=50  Lm=50  Saturation=[ 0,0 ; 0.0024,1.2 ; 1.0,1.52 ]  SpecifyInitialFlux=off  InitialFlux=0  BreakLoop=off  DiscreteSolver=Trapezoidal iterative  DataType=off  TransfoNumber=1
      settings: LibrarySourceBlock=|
      | sps_lib/Power Grid Elements/Multi-Winding
      | Transformer
  Multi-Winding Transformer9 : spsMultiWindingTransformerLib/Multi-Winding Transformer  LeftWindings=1  RightWindings=5  TappedWindings=no taps  NumberOfTaps=2  SetSaturation=off  Hysteresis=off  DataFile='hysteresis.mat'  Measurements=None  UNITS=pu  NominalPower=[P0 fn]  NominalVoltages="[ Source_Amp (1-sin(10/180*pi)/sin(50/180*pi))*2*sin(50/180*pi)*Ul_in sin(10/180*pi)/sin(50/180*pi)*2*sin(50/180*pi)*Ul_in  Ul_in (1-sin(10/180*pi)/sin(50/180*pi))*2*sin(50/180*pi)*Ul_in sin(10/180*pi)/sin(50/180*pi)*2*sin(50/180*pi)*Ul_in]"  WindingResistances="[ 0.005   0.005 0.005 0.005  0.005  0.005]"  WindingInductances="[ L_ori*5  L_sec L_sec L_sec L_sec L_sec]/5"  Rm=50  Lm=50  Saturation=[ 0,0 ; 0.0024,1.2 ; 1.0,1.52 ]  SpecifyInitialFlux=off  InitialFlux=0  BreakLoop=off  DiscreteSolver=Trapezoidal iterative  DataType=off  TransfoNumber=1
      settings: LibrarySourceBlock=|
      | sps_lib/Power Grid Elements/Multi-Winding
      | Transformer
  1+ : PMIOPort  Side=Left
  1+1 : PMIOPort  Port=2  Side=Left
  1+2 : PMIOPort  Port=3  Side=Left
  -20a : PMIOPort  Port=4  Side=Right
  -20b : PMIOPort  Port=5  Side=Right
  -20c : PMIOPort  Port=6  Side=Right
  0a : PMIOPort  Port=7  Side=Right
  0b : PMIOPort  Port=8  Side=Right
  0c : PMIOPort  Port=9  Side=Right
  +20a : PMIOPort  Port=10  Side=Right
  +20b : PMIOPort  Port=11  Side=Right
  +20c : PMIOPort  Port=12  Side=Right
  connections:
  Multi-Winding Transformer10/LConn2 -- Multi-Winding Transformer9/LConn2 -- Multi-Winding Transformer11/LConn2
  Multi-Winding Transformer11/RConn7 -- Multi-Winding Transformer10/RConn8 -- Multi-Winding Transformer11/RConn10
  Multi-Winding Transformer9/RConn1 -- Multi-Winding Transformer9/RConn4 -- Multi-Winding Transformer10/RConn2
  Multi-Winding Transformer10/RConn6 -- Multi-Winding Transformer9/RConn6 -- Multi-Winding Transformer11/RConn6
  Multi-Winding Transformer10/RConn7 -- Multi-Winding Transformer9/RConn8 -- Multi-Winding Transformer10/RConn10
  Multi-Winding Transformer11/RConn1 -- Multi-Winding Transformer9/RConn2 -- Multi-Winding Transformer11/RConn4
  Multi-Winding Transformer9/RConn10 -- Multi-Winding Transformer9/RConn7 -- Multi-Winding Transformer11/RConn8
  Multi-Winding Transformer10/RConn3 -- -20b/RConn1
  Multi-Winding Transformer10/RConn1 -- Multi-Winding Transformer10/RConn4 -- Multi-Winding Transformer11/RConn2
  Multi-Winding Transformer11/RConn3 -- -20c/RConn1
  Multi-Winding Transformer11/LConn1 -- 1+2/RConn1
  Multi-Winding Transformer11/RConn5 -- 0c/RConn1
  -20a/RConn1 -- Multi-Winding Transformer9/RConn3
  Multi-Winding Transformer9/RConn5 -- 0a/RConn1
  Multi-Winding Transformer10/LConn1 -- 1+1/RConn1
  +20a/RConn1 -- Multi-Winding Transformer9/RConn9
  Multi-Winding Transformer11/RConn9 -- +20c/RConn1
  Multi-Winding Transformer9/LConn1 -- 1+/RConn1
  Multi-Winding Transformer10/RConn5 -- 0b/RConn1
  Multi-Winding Transformer10/RConn9 -- +20b/RConn1

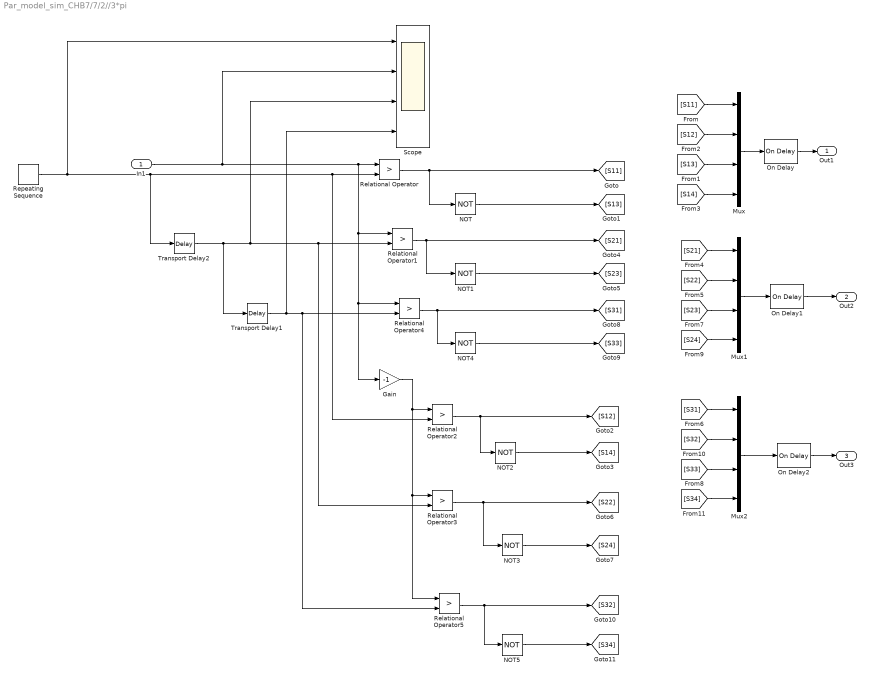
== system Par_model_sim_CHB7/7/2//3*pi ==
  In1 : Inport
  Gain : Gain  Gain=-1
  Mux : Mux
  Mux1 : Mux
  Mux2 : Mux
  NOT{,1..5} (6 alike) : Logic  Operator=NOT  AllPortsSameDT=off  OutDataTypeStr=boolean
  On Delay : spsOnDelayLib/On Delay  DelayType=On delay  delay=ttd  ic=0  Ts=0
  On Delay1 : spsOnDelayLib/On Delay  DelayType=On delay  delay=ttd  ic=0  Ts=0
  On Delay2 : spsOnDelayLib/On Delay  DelayType=On delay  delay=ttd  ic=0  Ts=0
  Relational Operator{,1..5} (6 alike) : RelationalOperator  Operator=>  OutDataTypeStr=boolean  RndMeth=Simplest  InputSameDT=off
  Repeating Sequence : simulink/Sources/Repeating Sequence  rep_seq_t=[0 0.5 1]/f_car  rep_seq_y=[-1 1 -1]*1000
  Scope : Scope  NumInputPorts=4
  Transport Delay1 : TransportDelay  DelayTime=tt/f_car  BufferSize=3072
  Transport Delay2 : TransportDelay  DelayTime=tt/f_car  BufferSize=3072
  Out1 : Outport
  Out2 : Outport  Port=2
  Out3 : Outport  Port=3
  wires:
  NOT/1 -> [S13]
  Transport Delay2/1 -> Scope/3, Relational Operator3/2, Relational Operator1/2, Transport Delay1/1
  [S14] -> Mux/4
  [S23] -> Mux1/3
  [S12] -> Mux/2
  In1/1 -> Scope/2, Relational Operator4/1, Gain/1, Relational Operator1/1, Relational Operator/1
  [S34] -> Mux2/4
  [S32] -> Mux2/2
  Mux2/1 -> On Delay2/1
  Relational Operator5/1 -> [S32], NOT5/1
  NOT2/1 -> [S14]
  [S21] -> Mux1/1
  NOT4/1 -> [S33]
  Relational Operator1/1 -> NOT1/1, [S21]
  [S22] -> Mux1/2
  [S33] -> Mux2/3
  NOT3/1 -> [S24]
  Mux/1 -> On Delay/1
  [S24] -> Mux1/4
  Relational Operator4/1 -> [S31], NOT4/1
  Gain/1 -> Relational Operator5/1, Relational Operator3/1, Relational Operator2/1
  [S13] -> Mux/3
  Relational Operator2/1 -> NOT2/1, [S12]
  [S31] -> Mux2/1
  [S11] -> Mux/1
  NOT5/1 -> [S34]
  Relational Operator/1 -> NOT/1, [S11]
  NOT1/1 -> [S23]
  Mux1/1 -> On Delay1/1
  Relational Operator3/1 -> NOT3/1, [S22]
  On Delay/1 -> Out1/1
  On Delay1/1 -> Out2/1
  On Delay2/1 -> Out3/1
  Transport Delay1/1 -> Scope/4, Relational Operator5/2, Relational Operator4/2
  Repeating Sequence/1 -> Scope/1, Transport Delay2/1, Relational Operator2/2, Relational Operator/2

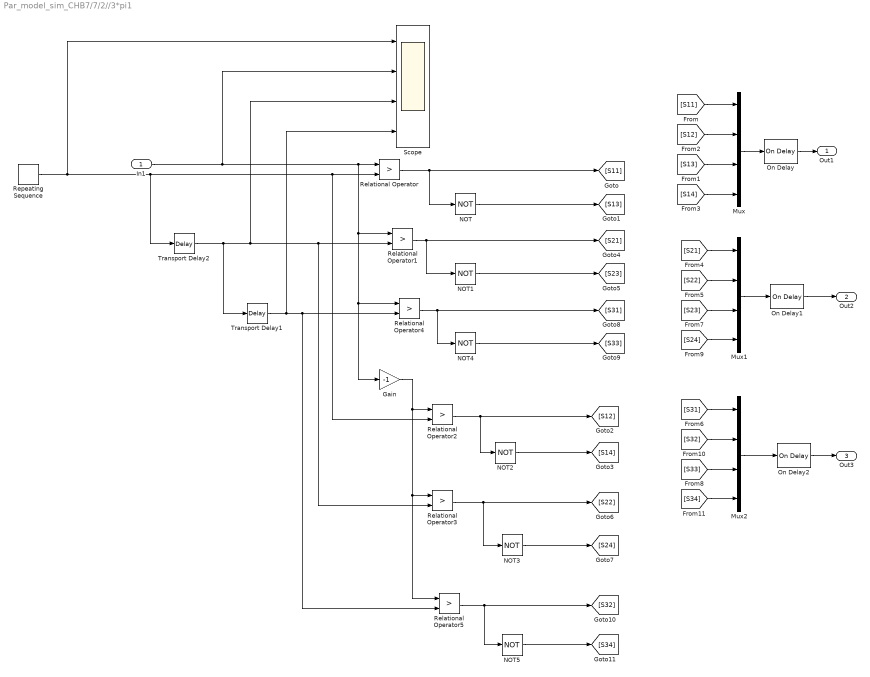
== system Par_model_sim_CHB7/7/2//3*pi1 ==
  In1 : Inport
  Gain : Gain  Gain=-1
  Mux : Mux
  Mux1 : Mux
  Mux2 : Mux
  NOT{,1..5} (6 alike) : Logic  Operator=NOT  AllPortsSameDT=off  OutDataTypeStr=boolean
  On Delay : spsOnDelayLib/On Delay  DelayType=On delay  delay=ttd  ic=0  Ts=0
  On Delay1 : spsOnDelayLib/On Delay  DelayType=On delay  delay=ttd  ic=0  Ts=0
  On Delay2 : spsOnDelayLib/On Delay  DelayType=On delay  delay=ttd  ic=0  Ts=0
  Relational Operator{,1..5} (6 alike) : RelationalOperator  Operator=>  OutDataTypeStr=boolean  RndMeth=Simplest  InputSameDT=off
  Repeating Sequence : simulink/Sources/Repeating Sequence  rep_seq_t=[0 0.5 1]/f_car  rep_seq_y=[-1 1 -1]*1000
  Scope : Scope  NumInputPorts=4
  Transport Delay1 : TransportDelay  DelayTime=tt/f_car  BufferSize=3072
  Transport Delay2 : TransportDelay  DelayTime=tt/f_car  BufferSize=3072
  Out1 : Outport
  Out2 : Outport  Port=2
  Out3 : Outport  Port=3
  wires:
  NOT/1 -> [S13]
  Transport Delay2/1 -> Scope/3, Relational Operator3/2, Relational Operator1/2, Transport Delay1/1
  [S14] -> Mux/4
  [S23] -> Mux1/3
  [S12] -> Mux/2
  In1/1 -> Scope/2, Relational Operator4/1, Gain/1, Relational Operator1/1, Relational Operator/1
  [S34] -> Mux2/4
  [S32] -> Mux2/2
  Mux2/1 -> On Delay2/1
  Relational Operator5/1 -> [S32], NOT5/1
  NOT2/1 -> [S14]
  [S21] -> Mux1/1
  NOT4/1 -> [S33]
  Relational Operator1/1 -> NOT1/1, [S21]
  [S22] -> Mux1/2
  [S33] -> Mux2/3
  NOT3/1 -> [S24]
  Mux/1 -> On Delay/1
  [S24] -> Mux1/4
  Relational Operator4/1 -> [S31], NOT4/1
  Gain/1 -> Relational Operator5/1, Relational Operator3/1, Relational Operator2/1
  [S13] -> Mux/3
  Relational Operator2/1 -> NOT2/1, [S12]
  [S31] -> Mux2/1
  [S11] -> Mux/1
  NOT5/1 -> [S34]
  Relational Operator/1 -> NOT/1, [S11]
  NOT1/1 -> [S23]
  Mux1/1 -> On Delay1/1
  Relational Operator3/1 -> NOT3/1, [S22]
  On Delay/1 -> Out1/1
  On Delay1/1 -> Out2/1
  On Delay2/1 -> Out3/1
  Transport Delay1/1 -> Scope/4, Relational Operator5/2, Relational Operator4/2
  Repeating Sequence/1 -> Scope/1, Transport Delay2/1, Relational Operator2/2, Relational Operator/2

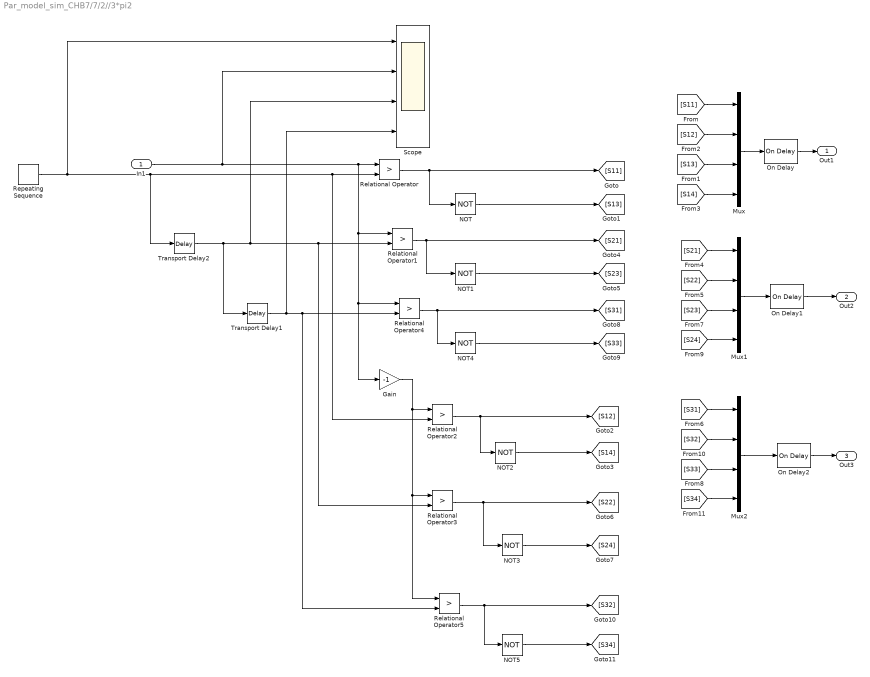
== system Par_model_sim_CHB7/7/2//3*pi2 ==
  In1 : Inport
  Gain : Gain  Gain=-1
  Mux : Mux
  Mux1 : Mux
  Mux2 : Mux
  NOT{,1..5} (6 alike) : Logic  Operator=NOT  AllPortsSameDT=off  OutDataTypeStr=boolean
  On Delay : spsOnDelayLib/On Delay  DelayType=On delay  delay=ttd  ic=0  Ts=0
  On Delay1 : spsOnDelayLib/On Delay  DelayType=On delay  delay=ttd  ic=0  Ts=0
  On Delay2 : spsOnDelayLib/On Delay  DelayType=On delay  delay=ttd  ic=0  Ts=0
  Relational Operator{,1..5} (6 alike) : RelationalOperator  Operator=>  OutDataTypeStr=boolean  RndMeth=Simplest  InputSameDT=off
  Repeating Sequence : simulink/Sources/Repeating Sequence  rep_seq_t=[0 0.5 1]/f_car  rep_seq_y=[-1 1 -1]*1000
  Scope : Scope  NumInputPorts=4
  Transport Delay1 : TransportDelay  DelayTime=tt/f_car  BufferSize=3072
  Transport Delay2 : TransportDelay  DelayTime=tt/f_car  BufferSize=3072
  Out1 : Outport
  Out2 : Outport  Port=2
  Out3 : Outport  Port=3
  wires:
  NOT/1 -> [S13]
  Transport Delay2/1 -> Scope/3, Relational Operator3/2, Relational Operator1/2, Transport Delay1/1
  [S14] -> Mux/4
  [S23] -> Mux1/3
  [S12] -> Mux/2
  In1/1 -> Scope/2, Relational Operator4/1, Gain/1, Relational Operator1/1, Relational Operator/1
  [S34] -> Mux2/4
  [S32] -> Mux2/2
  Mux2/1 -> On Delay2/1
  Relational Operator5/1 -> [S32], NOT5/1
  NOT2/1 -> [S14]
  [S21] -> Mux1/1
  NOT4/1 -> [S33]
  Relational Operator1/1 -> NOT1/1, [S21]
  [S22] -> Mux1/2
  [S33] -> Mux2/3
  NOT3/1 -> [S24]
  Mux/1 -> On Delay/1
  [S24] -> Mux1/4
  Relational Operator4/1 -> [S31], NOT4/1
  Gain/1 -> Relational Operator5/1, Relational Operator3/1, Relational Operator2/1
  [S13] -> Mux/3
  Relational Operator2/1 -> NOT2/1, [S12]
  [S31] -> Mux2/1
  [S11] -> Mux/1
  NOT5/1 -> [S34]
  Relational Operator/1 -> NOT/1, [S11]
  NOT1/1 -> [S23]
  Mux1/1 -> On Delay1/1
  Relational Operator3/1 -> NOT3/1, [S22]
  On Delay/1 -> Out1/1
  On Delay1/1 -> Out2/1
  On Delay2/1 -> Out3/1
  Transport Delay1/1 -> Scope/4, Relational Operator5/2, Relational Operator4/2
  Repeating Sequence/1 -> Scope/1, Transport Delay2/1, Relational Operator2/2, Relational Operator/2

== system Par_model_sim_CHB7/7/Subsystem ==
  In1 : Inport
  In2 : Inport  Port=2
  In3 : Inport  Port=3
  Add{1..3,9} (4 alike) : Sum
  Gain : Gain  Gain=-0.5
  Max : MinMax  Function=max  Inputs=3
  Max1 : MinMax  Inputs=3
  Out1 : Outport
  Out2 : Outport  Port=2
  Out3 : Outport  Port=3
  wires:
  In2/1 -> Add3/2, Max1/2, Max/2
  In3/1 -> Add9/2, Max1/3, Max/3
  In1/1 -> Max1/1, Add2/2, Max/1
  Gain/1 -> Add9/1, Add3/1, Add2/1
  Max/1 -> Add1/1
  Max1/1 -> Add1/2
  Add1/1 -> Gain/1
  Add9/1 -> Out3/1
  Add2/1 -> Out1/1
  Add3/1 -> Out2/1
